simulink model "model1"  (R2023a)
settings: Solver=VariableStepAuto  StartTime=0.0  StopTime=10.0  RelTol=1e-3
settings Model: Creator=vigro  LastModifiedBy=vigro

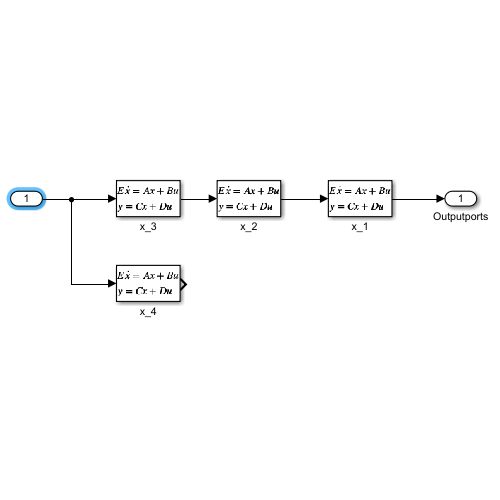
[thumbnail: Simulink's stored preview of the top-level diagram]
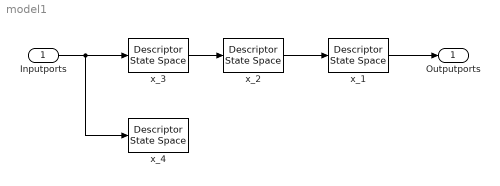
== system model1 ==
  Inputports : Inport
  x_{1..4} (4 alike) : DescriptorStateSpace  A=-2  C=0  D=0
  Outputports : Outport
  wires:
  x_3/1 -> x_2/1
  x_2/1 -> x_1/1
  Inputports/1 -> x_4/1, x_3/1
  x_1/1 -> Outputports/1
